simulink model "Simul1C"  (R2019b)
settings: Solver=VariableStepAuto  StartTime=0.0  StopTime=100  RelTol=1e-3
values from neighbouring files (symbols this model uses):
  A_n = 0.05 * pi / 180    (= 0.000872664625997)    [Proj1C.m]
  omega_n = 200    [Proj1C.m]
  w_lin = W    (= 0.0872)    [Proj1C.m]
libraries: cstblocks x2
settings Model: Creator=kmfrick  LastModifiedBy=kmfrick

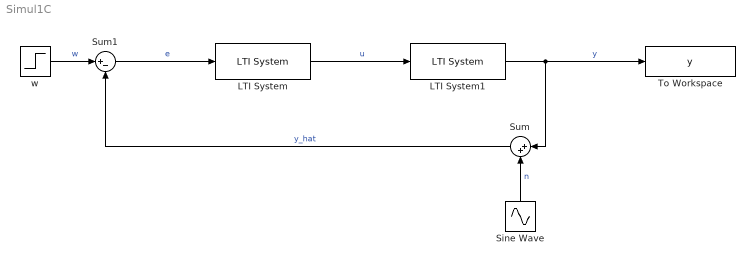
== system Simul1C ==
  LTI System : cstblocks/LTI System  sys=R_sim  IC=[]
  LTI System1 : cstblocks/LTI System  sys=G  IC=[]
  Sine Wave : Sin  Amplitude=A_n  Frequency=omega_n  SampleTime=0
  Sum : Sum  Inputs=|++
  Sum1 : Sum  Inputs=|+-
  To Workspace : ToWorkspace  VariableName=y  SaveFormat=Timeseries  SampleTime=-1
  w : Step  Time=pi/2  After=w_lin + pi/2  SampleTime=0
  wires:
  Sum/1 -> Sum1/2  "y_hat"
  Sine Wave/1 -> Sum/2  "n"
  w/1 -> Sum1/1  "w"
  LTI System1/1 -> Sum/1, To Workspace/1  "y"
  LTI System/1 -> LTI System1/1  "u"
  Sum1/1 -> LTI System/1  "e"
